simulink model "indmotorwithcc"  (R2021b)
settings: Solver=FixedStepAuto  StartTime=0.0  StopTime=1  FixedStep=1e-5  MinStep=1e-100  RelTol=1e-3
values from neighbouring files (symbols this model uses):
  Vdc = 300    [Induction_motor_parameter.m]
undefined symbols (not defined in the file or in its folder): A, alpha, Iqse_rated, Jm, Kac, Kas, Kic, Kpc, Kps, Kt, Lam_dre_rated, Lm, Lr, Ls, p, pp, Rr, Rs, sigma, Te_rated, Vs_rated, Ws
settings Model: Creator=lhjoon  LastModifiedBy=jun
settings SolverCC: AlgebraicLoopSolver=TrustRegion
settings DataIOCC: SaveFormat=Array  ReturnWorkspaceOutputs=off
settings DebuggingCC: SFMachineParentedDataDiag=warning
settings SFSimCC: CustomCodeUndefinedFunction=UseInterfaceOnly

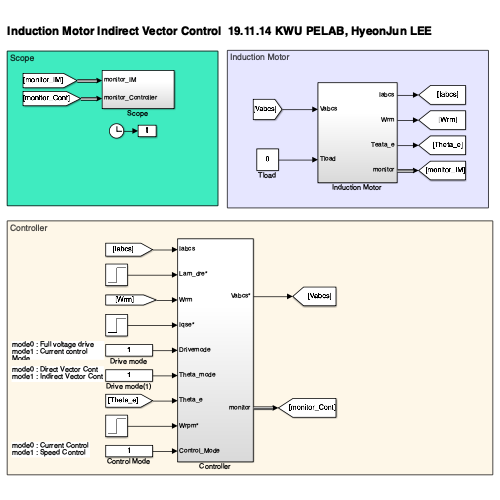
[thumbnail: Simulink's stored preview of the top-level diagram]
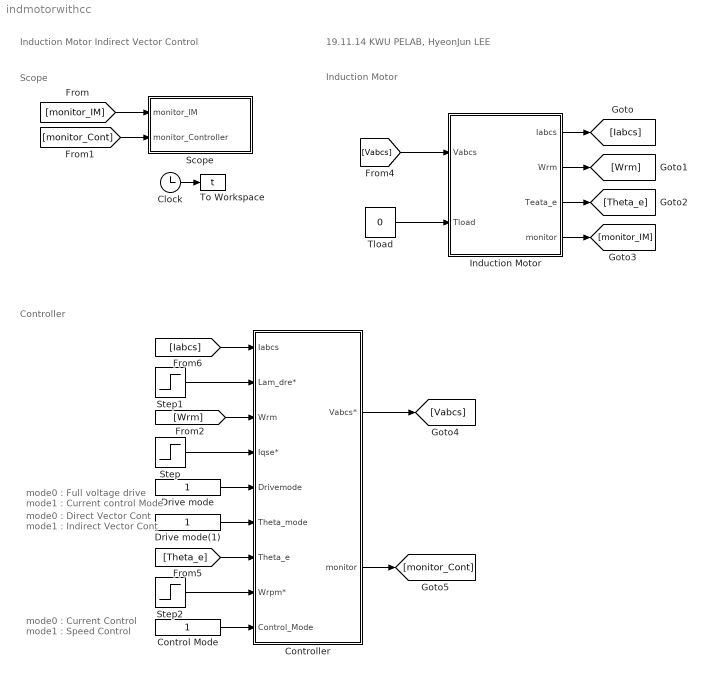
== system indmotorwithcc ==
  note: Controller
  note: mode0 : Full voltage drive
      | mode1 : Current control Mode
  note: Scope
  note: Induction Motor
  note: Induction Motor Indirect Vector Control
  note: mode0 : Direct Vector Cont
      | mode1 : Indirect Vector Cont
  note: 19.11.14 KWU PELAB, HyeonJun LEE
  note: mode0 : Current Control
      | mode1 : Speed Control
  Clock : Clock
  Control Mode : Constant
  Controller : Subsystem
  Drive mode : Constant
  Drive mode(1) : Constant
  Induction Motor : Subsystem
  Scope : Subsystem
  Step : Step  Time=0.2  After=8  SampleTime=0
  Step1 : Step  Time=0.1  After=Lam_dre_rated  SampleTime=0
  Step2 : Step  Time=0.3  After=1500  SampleTime=0
  "Tload " : Constant  Value=0
  To Workspace : ToWorkspace  VariableName=t  SampleTime=-1
  wires:
  Induction Motor/3(Teata_e) -> [Theta_e]
  Induction Motor/1(Iabcs) -> [Iabcs]
  Induction Motor/2(Wrm) -> [Wrm]
  Induction Motor/4(monitor) -> [monitor_IM]
  "Tload "/1 -> Induction Motor/2(Tload)
  Clock/1 -> To Workspace/1
  [monitor_IM] -> Scope/1(monitor_IM)
  [monitor_Cont] -> Scope/2(monitor_Controller)
  Controller/1(Vabcs*) -> [Vabcs]
  [Vabcs] -> Induction Motor/1(Vabcs)
  Drive mode/1 -> Controller/5(Drivemode)
  [Theta_e] -> Controller/7(Theta_e)
  [Iabcs] -> Controller/1(Iabcs)
  [Wrm] -> Controller/3(Wrm)
  Step1/1 -> Controller/2(Lam_dre*)
  Drive mode(1)/1 -> Controller/6(Theta_mode)
  Step/1 -> Controller/4(Iqse*)
  Controller/2(monitor) -> [monitor_Cont]
  Step2/1 -> Controller/8(Wrpm*)
  Control Mode/1 -> Controller/9(Control_Mode)

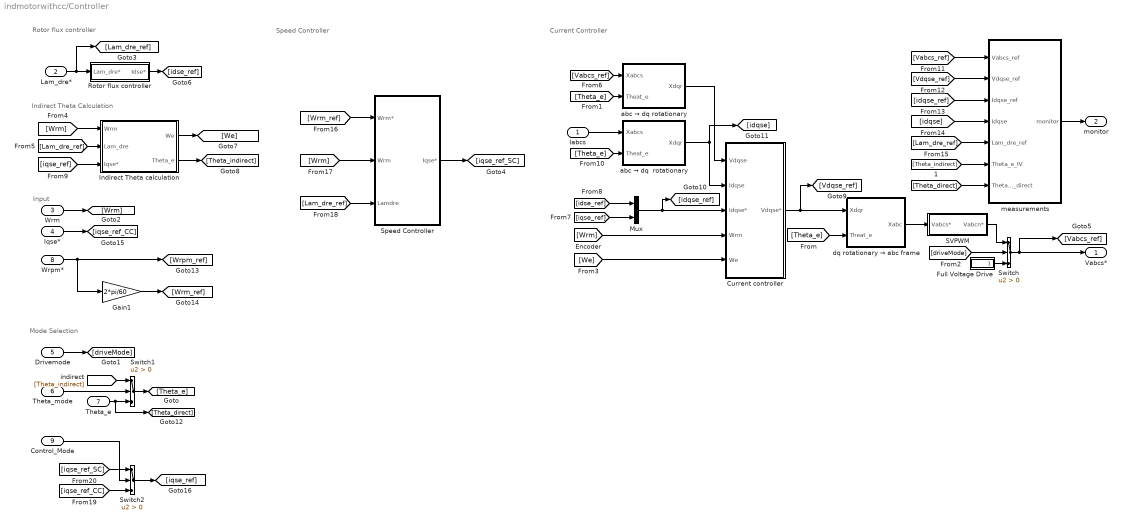
== system indmotorwithcc/Controller ==
  note: Mode Selection
  note: Speed Controller
  note: Current Controller
  note: Input
  note: Indirect Theta Calculation
  note: Rotor flux controller
  Iabcs : Inport
  Lam_dre* : Inport  Port=2
  Wrm : Inport  Port=3
  Iqse* : Inport  Port=4
  Drivemode : Inport  Port=5
  Theta_mode : Inport  Port=6
  Theta_e : Inport  Port=7
  Wrpm* : Inport  Port=8
  Control_Mode : Inport  Port=9
  "Current controller " : Subsystem
  Full Voltage Drive : Subsystem
  Gain1 : Gain  Gain=2*pi/60
  Indirect Theta calculation : Subsystem
  Mux : Mux  Inputs=2
  Rotor flux controller : Subsystem
  SVPWM : Subsystem
  Speed Controller : Subsystem
  Switch : Switch  Criteria=u2 > Threshold
  Switch1 : Switch  Criteria=u2 > Threshold
  Switch2 : Switch  Criteria=u2 > Threshold
  abc → dq  rotationary : Subsystem
  abc → dq rotationary : Subsystem
  dq rotationary → abc frame : Subsystem
  measurements : Subsystem
  Vabcs* : Outport  VectorParamsAs1DForOutWhenUnconnected=off
  monitor : Outport  Port=2  VectorParamsAs1DForOutWhenUnconnected=off
  wires:
  Full Voltage Drive/1(Vabcs) -> Switch/3
  [driveMode] -> Switch/2
  Switch/1 -> Vabcs*/1, [Vabcs_ref]
  dq rotationary → abc frame/1(Xabc) -> SVPWM/1(Vabcs*)
  Iabcs/1 -> abc → dq  rotationary/1(Xabcs)
  abc → dq  rotationary/1(Xdqr) -> [idqse], "Current controller "/2(Idqse)
  [Theta_e] -> dq rotationary → abc frame/2("Theat_e ")
  [Theta_e] -> abc → dq rotationary/2(Theat_e)
  abc → dq rotationary/1(Xdqr) -> "Current controller "/1(Vdqse)
  Drivemode/1 -> [driveMode]
  Wrm/1 -> [Wrm]
  [Wrm] -> "Current controller "/4(Wrm)
  Iqse*/1 -> [iqse_ref_CC]
  [We] -> "Current controller "/5(We)
  Lam_dre*/1 -> [Lam_dre_ref], Rotor flux controller/1(Lam_dre*)
  [Wrm] -> Indirect Theta calculation/1(Wrm)
  [Lam_dre_ref] -> Indirect Theta calculation/2(Lam_dre)
  Mux/1 -> [idqse_ref], "Current controller "/3(Idqse*)
  [Vabcs_ref] -> abc → dq rotationary/1(Xabcs)
  [idse_ref] -> Mux/1
  [iqse_ref] -> Mux/2
  Rotor flux controller/1(Idse*) -> [idse_ref]
  [iqse_ref] -> Indirect Theta calculation/3(Iqse*)
  Indirect Theta calculation/1(We) -> [We]
  Indirect Theta calculation/2(Theta_e) -> [Theta_indirect]
  Theta_mode/1 -> Switch1/2
  Switch1/1 -> [Theta_e]
  [Theta_indirect] -> Switch1/1
  Theta_e/1 -> [Theta_direct], Switch1/3
  [Theta_e] -> abc → dq  rotationary/2(Theat_e)
  measurements/1(monitor) -> monitor/1
  [Vabcs_ref] -> measurements/1(Vabcs_ref)
  "Current controller "/1(Vdqse*) -> [Vdqse_ref], dq rotationary → abc frame/1(Xdqr)
  [Vdqse_ref] -> measurements/2(Vdqse_ref)
  [idqse_ref] -> measurements/3(Idqse_ref)
  SVPWM/1(Vabcn*) -> Switch/1
  [idqse] -> measurements/4(Idqse)
  [Theta_indirect] -> measurements/6(Theta_e_IV)
  [Lam_dre_ref] -> measurements/5(Lam_dre_ref)
  [Theta_direct] -> measurements/7(Theta_e_direct)
  Wrpm*/1 -> Gain1/1, [Wrpm_ref]
  Gain1/1 -> [Wrm_ref]
  [Wrm_ref] -> Speed Controller/1(Wrm*)
  [Wrm] -> Speed Controller/2("Wrm ")
  [Lam_dre_ref] -> Speed Controller/3(Lamdre)
  Speed Controller/1(Iqse*) -> [iqse_ref_SC]
  Control_Mode/1 -> Switch2/2
  [iqse_ref_SC] -> Switch2/1
  [iqse_ref_CC] -> Switch2/3
  Switch2/1 -> [iqse_ref]

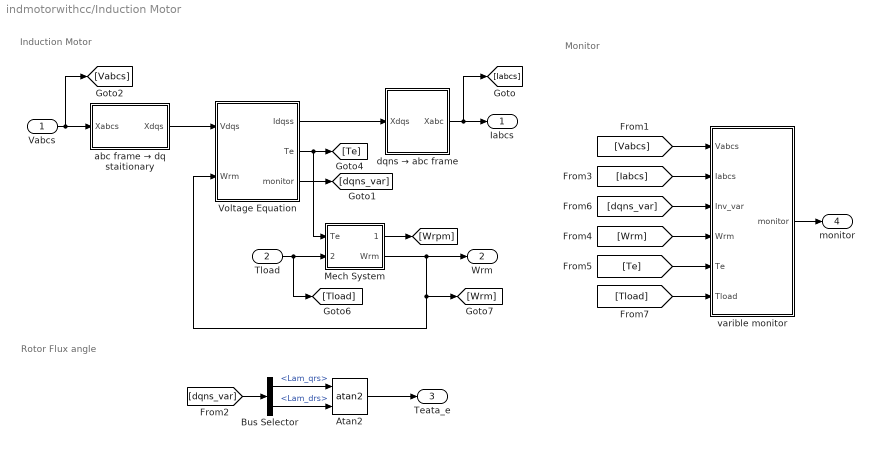
== system indmotorwithcc/Induction Motor ==
  note: Monitor
  note: Rotor Flux angle
  note: Induction Motor
  Vabcs : Inport
  Tload : Inport  Port=2
  Atan2 : Trigonometry  Operator=atan2
  Bus Selector : BusSelector  OutputSignals=Lam_qrs,Lam_drs
  Mech System : Subsystem
  Voltage Equation : Subsystem
  abc frame → dq staitionary : Subsystem
  dqns → abc frame : Subsystem
  varible monitor : Subsystem
  Iabcs : Outport  VectorParamsAs1DForOutWhenUnconnected=off
  Wrm : Outport  Port=2  VectorParamsAs1DForOutWhenUnconnected=off
  Teata_e : Outport  Port=3  VectorParamsAs1DForOutWhenUnconnected=off
  monitor : Outport  Port=4  VectorParamsAs1DForOutWhenUnconnected=off
  wires:
  Voltage Equation/3(monitor) -> [dqns_var]
  Voltage Equation/1(Idqss) -> dqns → abc frame/1(Xdqs)
  Bus Selector/2 -> Atan2/2  "<Lam_drs>"
  Atan2/1 -> Teata_e/1
  Bus Selector/1 -> Atan2/1  "<Lam_qrs>"
  Mech System/1(Wrpm) -> [Wrpm]
  Voltage Equation/2(Te) -> Mech System/1(Te), [Te]
  abc frame → dq staitionary/1(Xdqs) -> Voltage Equation/1(Vdqs)
  [dqns_var] -> Bus Selector/1
  Vabcs/1 -> [Vabcs], abc frame → dq staitionary/1(Xabcs)
  dqns → abc frame/1(Xabc) -> [Iabcs], Iabcs/1
  [Tload] -> varible monitor/6(Tload)
  [Te] -> varible monitor/5(Te)
  [Wrm] -> varible monitor/4(Wrm)
  [dqns_var] -> varible monitor/3(Inv_var)
  [Iabcs] -> varible monitor/2(Iabcs)
  [Vabcs] -> varible monitor/1(Vabcs)
  varible monitor/1(monitor) -> monitor/1
  Tload/1 -> [Tload], Mech System/2(TLoad)
  Mech System/2(Wrm) -> Voltage Equation/2(Wrm), [Wrm], Wrm/1

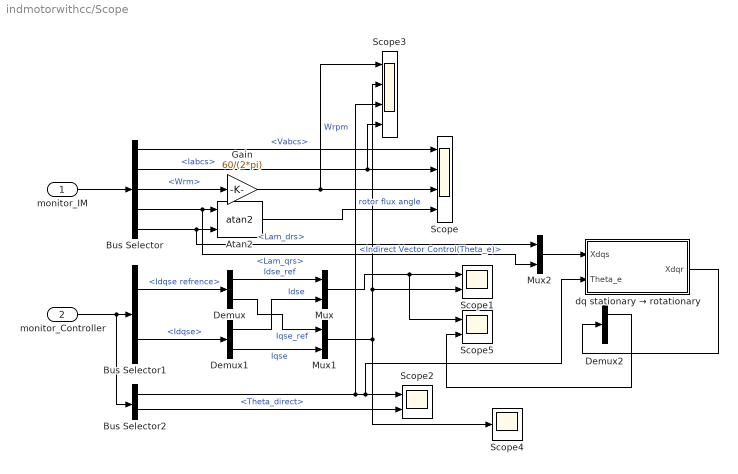
== system indmotorwithcc/Scope ==
  monitor_IM : Inport
  monitor_Controller : Inport  Port=2
  Atan2 : Trigonometry  Operator=atan2
  Bus Selector : BusSelector  OutputSignals=Electrical.3-phase.Vabcs,Electrical.3-phase.Iabcs,Mechanical.Wrm,Electrical.Stationary refrence frame.Lam_qrs,Electrical.Stationary refrence frame.Lam_drs
  Bus Selector1 : BusSelector  OutputSignals=Reference.Idqse refrence,Reference.Idqse
  Bus Selector2 : BusSelector  OutputSignals=Indirect Vector Control(Theta_e),Theta_direct
  Demux : Demux  Outputs=2
  Demux1 : Demux  Outputs=2
  Demux2 : Demux  Outputs=2
  Gain : Gain  Gain=60/(2*pi)
  Mux : Mux  Inputs=2
  Mux1 : Mux  Inputs=2
  Mux2 : Mux  Inputs=2
  Scope : Scope  NumInputPorts=4
  Scope1 : Scope  NumInputPorts=2
  Scope2 : Scope  NumInputPorts=2
  Scope3 : Scope  NumInputPorts=4
  Scope4 : Scope
  Scope5 : Scope  NumInputPorts=2
  dq stationary → rotationary : Subsystem
  wires:
  monitor_IM/1 -> Bus Selector/1
  Bus Selector/1 -> Scope/1  "<Vabcs>"
  Bus Selector/2 -> Scope3/4, Scope/2  "<Iabcs>"
  Bus Selector/3 -> Gain/1  "<Wrm>"
  Bus Selector/4 -> Mux2/2, Atan2/1  "<Lam_qrs>"
  Bus Selector/5 -> Mux2/1, Atan2/2  "<Lam_drs>"
  Atan2/1 -> Scope/4  "rotor flux angle"
  Gain/1 -> Scope3/1, Scope/3  "Wrpm"
  monitor_Controller/1 -> Bus Selector2/1, Bus Selector1/1
  Bus Selector1/1 -> Demux/1  "<Idqse refrence>"
  Bus Selector1/2 -> Demux1/1  "<Idqse>"
  Demux/1 -> Mux/1  "Idse_ref"
  Demux1/1 -> Mux/2  "Idse"
  Demux/2 -> Mux1/1  "Iqse_ref"
  Demux1/2 -> Mux1/2  "Iqse"
  Mux/1 -> Scope5/1, Scope1/1
  Mux1/1 -> Scope3/2, Scope1/2, Scope4/1
  Bus Selector2/1 -> Scope3/3, dq stationary → rotationary/2(Theta_e), Scope2/1  "<Indirect Vector Control(Theta_e)>"
  Bus Selector2/2 -> Scope2/2  "<Theta_direct>"
  Mux2/1 -> dq stationary → rotationary/1(Xdqs)
  dq stationary → rotationary/1(Xdqr) -> Demux2/1
  Demux2/1 -> Scope5/2

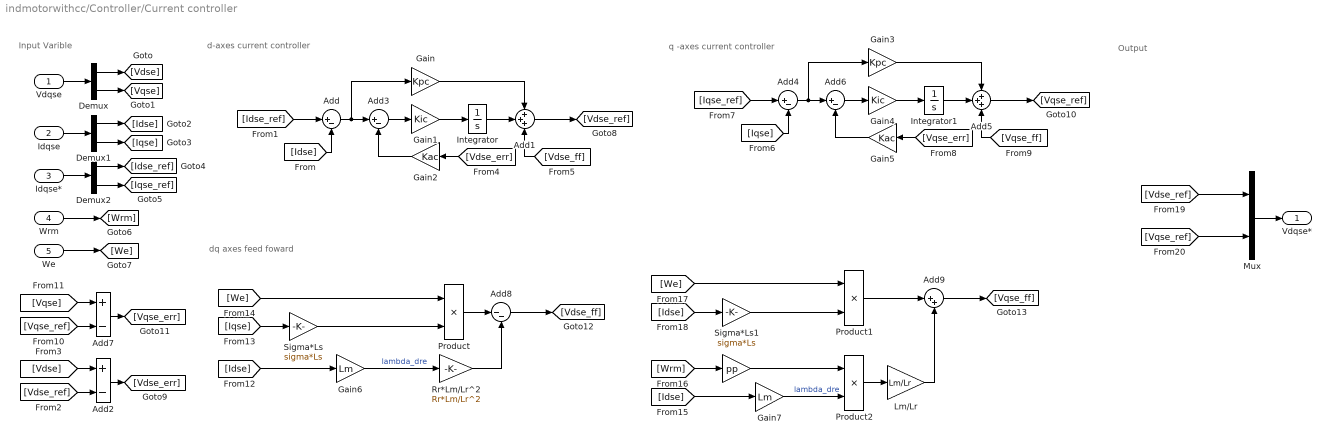
== system indmotorwithcc/Controller/Current controller  ==
  note: Output
  note: q -axes current controller
  note: d-axes current controller
  note: dq axes feed foward
  note: Input Varible
  Vdqse : Inport
  Idqse : Inport  Port=2
  Idqse* : Inport  Port=3
  Wrm : Inport  Port=4
  We : Inport  Port=5
  " " : Gain  Gain=pp
  Add{,3..4,6} (4 alike) : Sum  Inputs=|+-
  Add1 : Sum  Inputs=+++
  Add2 : Sum  Inputs=+-
  Add5 : Sum  Inputs=+++
  Add7 : Sum  Inputs=+-
  Add8 : Sum  Inputs=|--
  Add9 : Sum  Inputs=|++
  Demux : Demux  Outputs=2
  Demux1 : Demux  Outputs=2
  Demux2 : Demux  Outputs=2
  Gain : Gain  Gain=Kpc
  Gain1 : Gain  Gain=Kic
  Gain2 : Gain  Gain=Kac
  Gain3 : Gain  Gain=Kpc
  Gain4 : Gain  Gain=Kic
  Gain5 : Gain  Gain=Kac
  Gain6 : Gain  Gain=Lm
  Gain7 : Gain  Gain=Lm
  Integrator : Integrator
  Integrator1 : Integrator
  Lm/Lr : Gain  Gain=Lm/Lr
  Mux : Mux  Inputs=2
  Product : Product
  Product1 : Product
  Product2 : Product
  "Rr*Lm/Lr^2 " : Gain  Gain=Rr*Lm/Lr^2
  Sigma*Ls : Gain  Gain=sigma*Ls
  Sigma*Ls1 : Gain  Gain=sigma*Ls
  Vdqse* : Outport  VectorParamsAs1DForOutWhenUnconnected=off
  wires:
  Vdqse/1 -> Demux/1
  Demux/1 -> [Vdse]
  Demux/2 -> [Vqse]
  Demux1/1 -> [Idse]
  Idqse/1 -> Demux1/1
  Demux1/2 -> [Iqse]
  Demux2/1 -> [Idse_ref]
  Demux2/2 -> [Iqse_ref]
  Idqse*/1 -> Demux2/1
  Wrm/1 -> [Wrm]
  We/1 -> [We]
  [Idse] -> Add/2
  [Idse_ref] -> Add/1
  Add/1 -> Add3/1, Gain/1
  Gain1/1 -> Integrator/1
  Integrator/1 -> Add1/2
  Gain/1 -> Add1/1
  Add1/1 -> [Vdse_ref]
  [Vdse] -> Add2/1
  [Vdse_ref] -> Add2/2
  Add2/1 -> [Vdse_err]
  Add3/1 -> Gain1/1
  [Vdse_err] -> Gain2/1
  Gain2/1 -> Add3/2
  [Vdse_ff] -> Add1/3
  [Vqse_err] -> Gain5/1
  Gain5/1 -> Add6/2
  [Iqse] -> Add4/2
  Gain4/1 -> Integrator1/1
  Add6/1 -> Gain4/1
  Add4/1 -> Add6/1, Gain3/1
  Add5/1 -> [Vqse_ref]
  Gain3/1 -> Add5/1
  [Iqse_ref] -> Add4/1
  Integrator1/1 -> Add5/2
  [Vqse_ff] -> Add5/3
  [Vqse_ref] -> Add7/2
  Add7/1 -> [Vqse_err]
  [Vqse] -> Add7/1
  Add8/1 -> [Vdse_ff]
  "Rr*Lm/Lr^2 "/1 -> Add8/2
  [Idse] -> Gain6/1
  Gain6/1 -> "Rr*Lm/Lr^2 "/1  "lambda_dre"
  Product/1 -> Add8/1
  [Iqse] -> Sigma*Ls/1
  Sigma*Ls/1 -> Product/2
  [We] -> Product/1
  Product1/1 -> Add9/1
  Add9/1 -> [Vqse_ff]
  Lm/Lr/1 -> Add9/2
  Product2/1 -> Lm/Lr/1
  [Idse] -> Gain7/1
  Gain7/1 -> Product2/2  "lambda_dre"
  [Wrm] -> " "/1
  " "/1 -> Product2/1
  [We] -> Product1/1
  Sigma*Ls1/1 -> Product1/2
  [Idse] -> Sigma*Ls1/1
  Mux/1 -> Vdqse*/1
  [Vdse_ref] -> Mux/1
  [Vqse_ref] -> Mux/2

== system indmotorwithcc/Controller/Full Voltage Drive ==
  note: Full Voltage (RMS 220V)
  Mux : Mux  Inputs=3
  Vas : Sin  Amplitude=Vs_rated  Frequency=Ws  SampleTime=0
  Vbs : Sin  Amplitude=Vs_rated  Frequency=Ws  Phase=-2/3*pi  SampleTime=0
  Vcs : Sin  Amplitude=Vs_rated  Frequency=Ws  Phase=2/3*pi  SampleTime=0
  Vabcs : Outport  VectorParamsAs1DForOutWhenUnconnected=off
  wires:
  Vcs/1 -> Mux/3
  Vas/1 -> Mux/1
  Mux/1 -> Vabcs/1
  Vbs/1 -> Mux/2

== system indmotorwithcc/Controller/Indirect Theta calculation ==
  Wrm : Inport
  Lam_dre : Inport  Port=2
  Iqse* : Inport  Port=3
  Add : Sum  Inputs=|++
  Divide : Product  Inputs=*/
  Gain : Gain  Gain=pp
  Integrator : Subsystem
  Rr*Lm/Lr : Gain  Gain=Lm/Lr*Rr
  Saturation4 : Saturate  UpperLimit=inf  LowerLimit=1e-04
  We : Outport  VectorParamsAs1DForOutWhenUnconnected=off
  Theta_e : Outport  Port=2  VectorParamsAs1DForOutWhenUnconnected=off
  wires:
  Iqse*/1 -> Rr*Lm/Lr/1
  Lam_dre/1 -> Saturation4/1
  Saturation4/1 -> Divide/2
  Rr*Lm/Lr/1 -> Divide/1
  Divide/1 -> Add/1  "Wsl"
  Wrm/1 -> Gain/1
  Gain/1 -> Add/2  "Wr"
  Add/1 -> Integrator/1(We), We/1
  Integrator/1(Theta_e) -> Theta_e/1

== system indmotorwithcc/Controller/Rotor flux controller ==
  Lam_dre* : Inport
  Gain : Gain  Gain=1/Lm
  Idse* : Outport  VectorParamsAs1DForOutWhenUnconnected=off
  wires:
  Gain/1 -> Idse*/1
  Lam_dre*/1 -> Gain/1

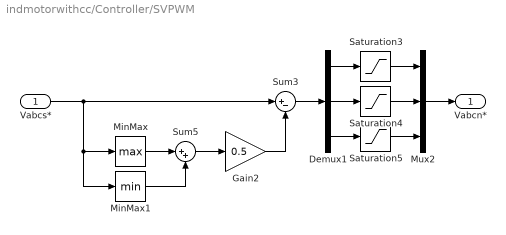
== system indmotorwithcc/Controller/SVPWM ==
  Vabcs* : Inport
  Demux1 : Demux  Outputs=3
  Gain2 : Gain  Gain=0.5
  MinMax : MinMax  Function=max
  MinMax1 : MinMax
  Mux2 : Mux  Inputs=3
  Saturation3 : Saturate  UpperLimit=Vdc/2  LowerLimit=-Vdc/2
  Saturation4 : Saturate  UpperLimit=Vdc/2  LowerLimit=-Vdc/2
  Saturation5 : Saturate  UpperLimit=Vdc/2  LowerLimit=-Vdc/2
  Sum3 : Sum  Inputs=|+-
  Sum5 : Sum  Inputs=|++
  Vabcn* : Outport  VectorParamsAs1DForOutWhenUnconnected=off
  wires:
  Vabcs*/1 -> Sum3/1, MinMax1/1, MinMax/1
  MinMax/1 -> Sum5/1
  Sum5/1 -> Gain2/1
  MinMax1/1 -> Sum5/2
  Gain2/1 -> Sum3/2
  Demux1/1 -> Saturation3/1
  Demux1/2 -> Saturation4/1
  Demux1/3 -> Saturation5/1
  Sum3/1 -> Demux1/1
  Saturation3/1 -> Mux2/1
  Saturation4/1 -> Mux2/2
  Saturation5/1 -> Mux2/3
  Mux2/1 -> Vabcn*/1

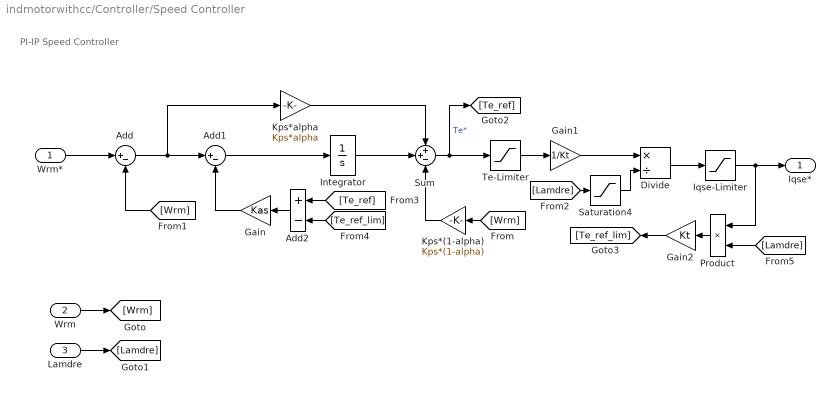
== system indmotorwithcc/Controller/Speed Controller ==
  note: PI-IP Speed Controller
  Wrm* : Inport
  "Wrm " : Inport  Port=2
  Lamdre : Inport  Port=3
  Add : Sum  Inputs=|+-
  Add1 : Sum  Inputs=|+-
  Add2 : Sum  Inputs=+-
  Divide : Product  Inputs=*/
  Gain : Gain  Gain=Kas
  Gain1 : Gain  Gain=1/Kt
  Gain2 : Gain  Gain=Kt
  Integrator : Integrator
  Iqse-Limiter : Saturate  UpperLimit=Iqse_rated  LowerLimit=-Iqse_rated
  Kps*(1-alpha) : Gain  Gain=Kps*(1-alpha)
  Kps*alpha : Gain  Gain=Kps*alpha
  Product : Product
  Saturation4 : Saturate  UpperLimit=inf  LowerLimit=1e-04
  Sum : Sum  Inputs=++-
  Te-Limiter : Saturate  UpperLimit=Te_rated  LowerLimit=-Te_rated
  Iqse* : Outport  VectorParamsAs1DForOutWhenUnconnected=off
  wires:
  Wrm*/1 -> Add/1
  "Wrm "/1 -> [Wrm]
  Lamdre/1 -> [Lamdre]
  Add/1 -> Kps*alpha/1, Add1/1
  Gain/1 -> Add1/2
  Add1/1 -> Integrator/1
  Integrator/1 -> Sum/2
  Kps*(1-alpha)/1 -> Sum/3
  Kps*alpha/1 -> Sum/1
  [Wrm] -> Add/2
  [Wrm] -> Kps*(1-alpha)/1
  Add2/1 -> Gain/1
  Sum/1 -> Te-Limiter/1, [Te_ref]  "Te*"
  Te-Limiter/1 -> Gain1/1
  Gain1/1 -> Divide/1
  Divide/1 -> Iqse-Limiter/1
  Iqse-Limiter/1 -> Iqse*/1, Product/1
  [Te_ref] -> Add2/1
  [Te_ref_lim] -> Add2/2
  [Lamdre] -> Product/2
  Gain2/1 -> [Te_ref_lim]
  Product/1 -> Gain2/1
  Saturation4/1 -> Divide/2
  [Lamdre] -> Saturation4/1

== system indmotorwithcc/Controller/abc → dq  rotationary ==
  Xabcs : Inport
  Theat_e : Inport  Port=2
  abc frame → dq staitionary : Subsystem
  dq stationary → rotationary : Subsystem
  Xdqr : Outport  VectorParamsAs1DForOutWhenUnconnected=off
  wires:
  Xabcs/1 -> abc frame → dq staitionary/1(Xabcs)
  abc frame → dq staitionary/1(Xdqs) -> dq stationary → rotationary/1(Xdqs)
  Theat_e/1 -> dq stationary → rotationary/2(Theta_e)
  dq stationary → rotationary/1(Xdqr) -> Xdqr/1

== system indmotorwithcc/Controller/abc → dq rotationary ==
  Xabcs : Inport
  Theat_e : Inport  Port=2
  abc frame → dq staitionary : Subsystem
  dq stationary → rotationary : Subsystem
  Xdqr : Outport  VectorParamsAs1DForOutWhenUnconnected=off
  wires:
  Xabcs/1 -> abc frame → dq staitionary/1(Xabcs)
  abc frame → dq staitionary/1(Xdqs) -> dq stationary → rotationary/1(Xdqs)
  Theat_e/1 -> dq stationary → rotationary/2(Theta_e)
  dq stationary → rotationary/1(Xdqr) -> Xdqr/1

== system indmotorwithcc/Controller/dq rotationary → abc frame ==
  Xdqr : Inport
  "Theat_e " : Inport  Port=2
  dq rotatinoary → dq stationary : Subsystem
  dq stationary → abc frame : Subsystem
  Xabc : Outport  VectorParamsAs1DForOutWhenUnconnected=off
  wires:
  "Theat_e "/1 -> dq rotatinoary → dq stationary/2(Theta_e)
  Xdqr/1 -> dq rotatinoary → dq stationary/1(Xdqr)
  dq rotatinoary → dq stationary/1(Xdqs) -> dq stationary → abc frame/1(Xdqs)
  dq stationary → abc frame/1(Xabc) -> Xabc/1

== system indmotorwithcc/Controller/measurements ==
  Vabcs_ref : Inport
  Vdqse_ref : Inport  Port=2
  Idqse_ref : Inport  Port=3
  Idqse : Inport  Port=4
  Lam_dre_ref : Inport  Port=5
  Theta_e_IV : Inport  Port=6
  Theta_e_direct : Inport  Port=7
  Bus Creator1 : BusCreator  Inputs=2
  Bus Creator2 : BusCreator  Inputs=4
  Bus Creator4 : BusCreator  Inputs=3
  monitor : Outport  VectorParamsAs1DForOutWhenUnconnected=off
  wires:
  Theta_e_IV/1 -> Bus Creator4/2  "Indirect Vector Control(Theta_e)"
  Idqse_ref/1 -> Bus Creator2/2  "Idqse refrence"
  Bus Creator4/1 -> monitor/1
  Bus Creator2/1 -> Bus Creator4/1  "Reference"
  Bus Creator1/1 -> Bus Creator2/1  "Voltage reference"
  Lam_dre_ref/1 -> Bus Creator2/4  "Lam_dre_ref"
  Vdqse_ref/1 -> Bus Creator1/2  "Vdqse_ref"
  Vabcs_ref/1 -> Bus Creator1/1  "Vabcs_ref"
  Idqse/1 -> Bus Creator2/3  "Idqse"
  Theta_e_direct/1 -> Bus Creator4/3  "Theta_direct"

== system indmotorwithcc/Induction Motor/Mech System ==
  note: Mech System
  Te : Inport
  TLoad : Inport  Port=2
  Add : Sum  Inputs=+-
  Gain : Gain  Gain=1/Jm
  Gain1 : Gain  Gain=60/(2*pi)
  Integrator : Integrator
  Wrpm : Outport  VectorParamsAs1DForOutWhenUnconnected=off
  Wrm : Outport  Port=2  VectorParamsAs1DForOutWhenUnconnected=off
  wires:
  Integrator/1 -> Gain1/1, Wrm/1
  Gain/1 -> Integrator/1
  Te/1 -> Add/1
  Add/1 -> Gain/1
  TLoad/1 -> Add/2
  Gain1/1 -> Wrpm/1

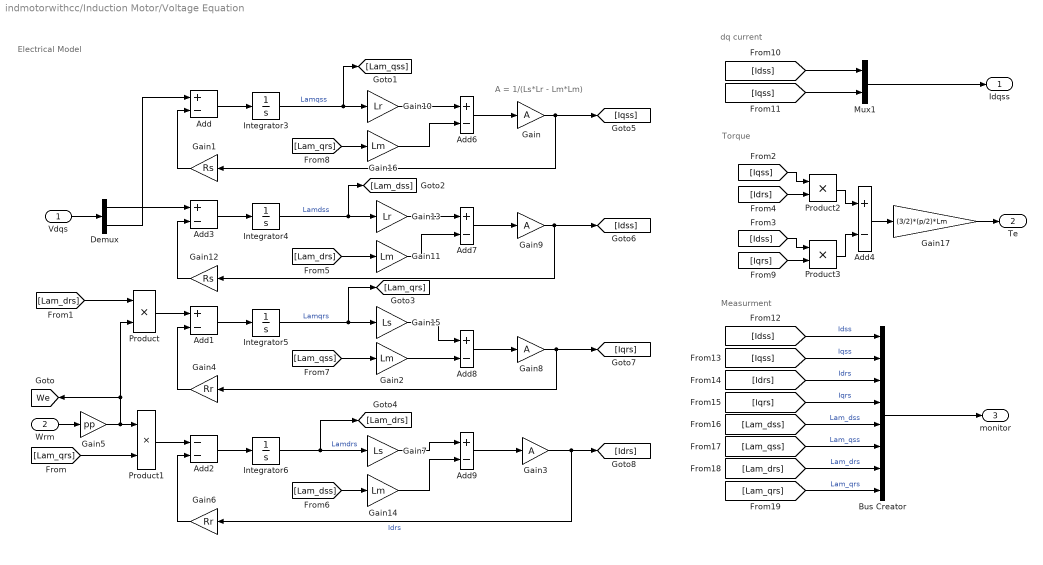
== system indmotorwithcc/Induction Motor/Voltage Equation ==
  note: Measurment
  note: dq current
  note: Torque
  note: Electrical Model
  note: A = 1/(Ls*Lr - Lm*Lm)
  Vdqs : Inport
  Wrm : Inport  Port=2
  Add{,1,3..4,6..9} (8 alike) : Sum  Inputs=+-
  Add2 : Sum  Inputs=--
  Bus Creator : BusCreator  Inputs=8
  Demux : Demux  Outputs=2
  Gain{,3,8..9} (4 alike) : Gain  Gain=A
  Gain1 : Gain  Gain=Rs
  Gain10 : Gain  Gain=Lr
  Gain{2,11,14,16} (4 alike) : Gain  Gain=Lm
  Gain12 : Gain  Gain=Rs
  Gain13 : Gain  Gain=Lr
  Gain15 : Gain  Gain=Ls
  Gain17 : Gain  Gain=(3/2)*(p/2)*Lm
  Gain4 : Gain  Gain=Rr
  Gain5 : Gain  Gain=pp
  Gain6 : Gain  Gain=Rr
  Gain7 : Gain  Gain=Ls
  Integrator{3..6} (4 alike) : Integrator
  Mux1 : Mux  Inputs=2
  Product{,1..3} (4 alike) : Product
  Idqss : Outport  VectorParamsAs1DForOutWhenUnconnected=off
  Te : Outport  Port=2  VectorParamsAs1DForOutWhenUnconnected=off
  monitor : Outport  Port=3  VectorParamsAs1DForOutWhenUnconnected=off
  tag scope: We=global
  wires:
  Gain/1 -> Gain1/1, [Iqss]
  Wrm/1 -> Gain5/1
  Integrator3/1 -> [Lam_qss], Gain10/1  "Lamqss"
  Integrator4/1 -> [Lam_dss], Gain13/1  "Lamdss"
  Integrator5/1 -> [Lam_qrs], Gain15/1  "Lamqrs"
  Integrator6/1 -> [Lam_drs], Gain7/1  "Lamdrs"
  Gain9/1 -> Gain12/1, [Idss]
  Gain8/1 -> [Iqrs], Gain4/1
  Gain3/1 -> [Idrs], Gain6/1  "Idrs"
  Add6/1 -> Gain/1
  Add7/1 -> Gain9/1
  Add8/1 -> Gain8/1
  Add9/1 -> Gain3/1
  Gain10/1 -> Add6/1
  Add/1 -> Integrator3/1
  Gain1/1 -> Add/2
  Add1/1 -> Integrator5/1
  Gain4/1 -> Add1/2
  Product/1 -> Add1/1
  Gain5/1 -> Product/2, [We], Product1/1
  Add2/1 -> Integrator6/1
  Gain6/1 -> Add2/2
  Gain7/1 -> Add9/1
  Add3/1 -> Integrator4/1
  Gain12/1 -> Add3/2
  Gain13/1 -> Add7/1
  Product1/1 -> Add2/1
  Demux/2 -> Add/1
  Gain17/1 -> Te/1
  Add4/1 -> Gain17/1
  Product2/1 -> Add4/1
  Product3/1 -> Add4/2
  [Lam_qrs] -> Product1/2
  [Lam_drs] -> Product/1
  [Iqss] -> Product2/1
  [Idss] -> Product3/1
  [Iqrs] -> Product3/2
  Gain11/1 -> Add7/2
  [Lam_drs] -> Gain11/1
  [Lam_dss] -> Gain14/1
  Gain16/1 -> Add6/2
  [Lam_qss] -> Gain2/1
  Gain15/1 -> Add8/1
  Gain2/1 -> Add8/2
  [Lam_qrs] -> Gain16/1
  [Idrs] -> Product2/2
  Gain14/1 -> Add9/2
  [Idss] -> Mux1/1
  [Iqss] -> Mux1/2
  Mux1/1 -> Idqss/1
  [Idss] -> Bus Creator/1  "Idss"
  [Iqss] -> Bus Creator/2  "Iqss"
  [Idrs] -> Bus Creator/3  "Idrs"
  [Iqrs] -> Bus Creator/4  "Iqrs"
  [Lam_dss] -> Bus Creator/5  "Lam_dss"
  [Lam_qss] -> Bus Creator/6  "Lam_qss"
  [Lam_drs] -> Bus Creator/7  "Lam_drs"
  [Lam_qrs] -> Bus Creator/8  "Lam_qrs"
  Bus Creator/1 -> monitor/1
  Vdqs/1 -> Demux/1
  Demux/1 -> Add3/1

== system indmotorwithcc/Induction Motor/abc frame → dq staitionary ==
  Xabcs : Inport
  Add : Sum  Inputs=+--
  Add1 : Sum  Inputs=+-
  Demux : Demux  Outputs=3
  Gain : Gain  Gain=2
  Gain1 : Gain  Gain=1/3
  Gain2 : Gain  Gain=1/sqrt(3)
  Mux : Mux  Inputs=2
  Xdqs : Outport  VectorParamsAs1DForOutWhenUnconnected=off
  wires:
  Demux/1 -> Gain/1
  Gain/1 -> Add/1
  Demux/2 -> Add1/1, Add/2
  Demux/3 -> Add1/2, Add/3
  Add/1 -> Gain1/1
  Gain1/1 -> Mux/1
  Gain2/1 -> Mux/2
  Add1/1 -> Gain2/1
  Mux/1 -> Xdqs/1
  Xabcs/1 -> Demux/1

== system indmotorwithcc/Induction Motor/dqns → abc frame ==
  Xdqs : Inport
  Add : Sum  Inputs=-+
  Add1 : Sum  Inputs=--
  Demux : Demux  Outputs=2
  Gain : Gain  Gain=1/2
  Gain1 : Gain  Gain=sqrt(3)/2
  Mux : Mux  Inputs=3
  Xabc : Outport  VectorParamsAs1DForOutWhenUnconnected=off
  wires:
  Demux/1 -> Mux/1, Gain/1
  Add/1 -> Mux/2
  Add1/1 -> Mux/3
  Demux/2 -> Gain1/1
  Gain1/1 -> Add1/2, Add/2
  Gain/1 -> Add1/1, Add/1
  Mux/1 -> Xabc/1
  Xdqs/1 -> Demux/1

== system indmotorwithcc/Induction Motor/varible monitor ==
  Vabcs : Inport
  Iabcs : Inport  Port=2
  Inv_var : Inport  Port=3
  Wrm : Inport  Port=4
  Te : Inport  Port=5
  Tload : Inport  Port=6
  Bus Creator1 : BusCreator  Inputs=2
  Bus Creator2 : BusCreator  Inputs=2
  Bus Creator3 : BusCreator  Inputs=4
  Bus Creator4 : BusCreator  Inputs=2
  Gain5 : Gain  Gain=pp
  monitor : Outport  VectorParamsAs1DForOutWhenUnconnected=off
  wires:
  Vabcs/1 -> Bus Creator1/1  "Vabcs"
  Iabcs/1 -> Bus Creator1/2  "Iabcs"
  Bus Creator4/1 -> monitor/1
  Bus Creator1/1 -> Bus Creator2/1  "3-phase"
  Inv_var/1 -> Bus Creator2/2  "Stationary refrence frame"
  Wrm/1 -> Gain5/1, Bus Creator3/1  "Wrm"
  Te/1 -> Bus Creator3/3
  Bus Creator3/1 -> Bus Creator4/2  "Mechanical"
  Bus Creator2/1 -> Bus Creator4/1  "Electrical"
  Gain5/1 -> Bus Creator3/2  "Wr"
  Tload/1 -> Bus Creator3/4

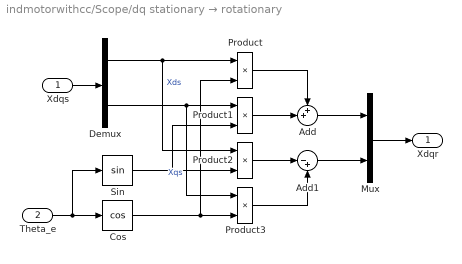
== system indmotorwithcc/Scope/dq stationary → rotationary ==
  Xdqs : Inport
  Theta_e : Inport  Port=2
  Add : Sum  Inputs=++|
  Add1 : Sum  Inputs=|-+
  Cos : Trigonometry  Operator=cos
  Demux : Demux  Outputs=2
  Mux : Mux  Inputs=2
  Product{,1..3} (4 alike) : Product
  Sin : Trigonometry
  Xdqr : Outport  VectorParamsAs1DForOutWhenUnconnected=off
  wires:
  Xdqs/1 -> Demux/1
  Demux/1 -> Product2/1, Product/1  "Xds"
  Demux/2 -> Product3/1, Product1/1  "Xqs"
  Theta_e/1 -> Sin/1, Cos/1
  Cos/1 -> Product3/2, Product/2
  Product/1 -> Add/1
  Product1/1 -> Add/2
  Product2/1 -> Add1/1
  Product3/1 -> Add1/2
  Add1/1 -> Mux/2
  Add/1 -> Mux/1
  Sin/1 -> Product2/2, Product1/2
  Mux/1 -> Xdqr/1

== system indmotorwithcc/Controller/Indirect Theta calculation/Integrator ==
  We : Inport
  Integrator : Integrator
  bound pi : Subsystem
  Theta_e : Outport  VectorParamsAs1DForOutWhenUnconnected=off
  wires:
  We/1 -> Integrator/1
  Integrator/1 -> bound pi/1(theta)
  bound pi/1(bounded_theta) -> Theta_e/1

== system indmotorwithcc/Controller/abc → dq  rotationary/abc frame → dq staitionary ==
  Xabcs : Inport
  Add : Sum  Inputs=+--
  Add1 : Sum  Inputs=+-
  Demux : Demux  Outputs=3
  Gain : Gain  Gain=2
  Gain1 : Gain  Gain=1/3
  Gain2 : Gain  Gain=1/sqrt(3)
  Mux : Mux  Inputs=2
  Xdqs : Outport  VectorParamsAs1DForOutWhenUnconnected=off
  wires:
  Demux/1 -> Gain/1
  Gain/1 -> Add/1
  Demux/2 -> Add1/1, Add/2
  Demux/3 -> Add1/2, Add/3
  Add/1 -> Gain1/1
  Gain1/1 -> Mux/1
  Gain2/1 -> Mux/2
  Add1/1 -> Gain2/1
  Mux/1 -> Xdqs/1
  Xabcs/1 -> Demux/1

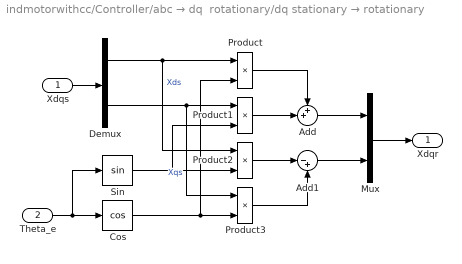
== system indmotorwithcc/Controller/abc → dq  rotationary/dq stationary → rotationary ==
  Xdqs : Inport
  Theta_e : Inport  Port=2
  Add : Sum  Inputs=++|
  Add1 : Sum  Inputs=|-+
  Cos : Trigonometry  Operator=cos
  Demux : Demux  Outputs=2
  Mux : Mux  Inputs=2
  Product{,1..3} (4 alike) : Product
  Sin : Trigonometry
  Xdqr : Outport  VectorParamsAs1DForOutWhenUnconnected=off
  wires:
  Xdqs/1 -> Demux/1
  Demux/1 -> Product2/1, Product/1  "Xds"
  Demux/2 -> Product3/1, Product1/1  "Xqs"
  Theta_e/1 -> Sin/1, Cos/1
  Cos/1 -> Product3/2, Product/2
  Product/1 -> Add/1
  Product1/1 -> Add/2
  Product2/1 -> Add1/1
  Product3/1 -> Add1/2
  Add1/1 -> Mux/2
  Add/1 -> Mux/1
  Sin/1 -> Product2/2, Product1/2
  Mux/1 -> Xdqr/1

== system indmotorwithcc/Controller/abc → dq rotationary/abc frame → dq staitionary ==
  Xabcs : Inport
  Add : Sum  Inputs=+--
  Add1 : Sum  Inputs=+-
  Demux : Demux  Outputs=3
  Gain : Gain  Gain=2
  Gain1 : Gain  Gain=1/3
  Gain2 : Gain  Gain=1/sqrt(3)
  Mux : Mux  Inputs=2
  Xdqs : Outport  VectorParamsAs1DForOutWhenUnconnected=off
  wires:
  Demux/1 -> Gain/1
  Gain/1 -> Add/1
  Demux/2 -> Add1/1, Add/2
  Demux/3 -> Add1/2, Add/3
  Add/1 -> Gain1/1
  Gain1/1 -> Mux/1
  Gain2/1 -> Mux/2
  Add1/1 -> Gain2/1
  Mux/1 -> Xdqs/1
  Xabcs/1 -> Demux/1

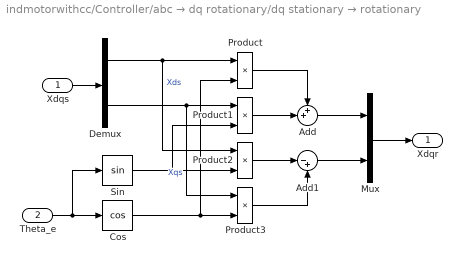
== system indmotorwithcc/Controller/abc → dq rotationary/dq stationary → rotationary ==
  Xdqs : Inport
  Theta_e : Inport  Port=2
  Add : Sum  Inputs=++|
  Add1 : Sum  Inputs=|-+
  Cos : Trigonometry  Operator=cos
  Demux : Demux  Outputs=2
  Mux : Mux  Inputs=2
  Product{,1..3} (4 alike) : Product
  Sin : Trigonometry
  Xdqr : Outport  VectorParamsAs1DForOutWhenUnconnected=off
  wires:
  Xdqs/1 -> Demux/1
  Demux/1 -> Product2/1, Product/1  "Xds"
  Demux/2 -> Product3/1, Product1/1  "Xqs"
  Theta_e/1 -> Sin/1, Cos/1
  Cos/1 -> Product3/2, Product/2
  Product/1 -> Add/1
  Product1/1 -> Add/2
  Product2/1 -> Add1/1
  Product3/1 -> Add1/2
  Add1/1 -> Mux/2
  Add/1 -> Mux/1
  Sin/1 -> Product2/2, Product1/2
  Mux/1 -> Xdqr/1

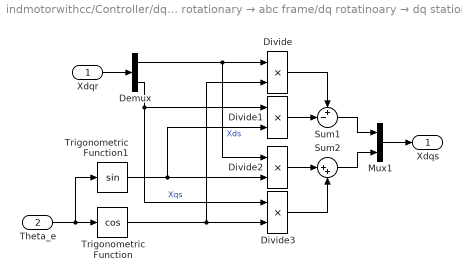
== system indmotorwithcc/Controller/dq rotationary → abc frame/dq rotatinoary → dq stationary ==
  Xdqr : Inport
  Theta_e : Inport  Port=2
  Demux : Demux  Outputs=2
  Divide{,1..3} (4 alike) : Product  Inputs=**
  Mux1 : Mux  Inputs=2
  Sum1 : Sum  Inputs=+-|
  Sum2 : Sum  Inputs=|++
  Trigonometric Function : Trigonometry  Operator=cos
  Trigonometric Function1 : Trigonometry
  Xdqs : Outport  VectorParamsAs1DForOutWhenUnconnected=off
  wires:
  Xdqr/1 -> Demux/1
  Mux1/1 -> Xdqs/1
  Divide3/1 -> Sum2/2
  Sum2/1 -> Mux1/2
  Divide2/1 -> Sum2/1
  Divide/1 -> Sum1/1
  Sum1/1 -> Mux1/1
  Divide1/1 -> Sum1/2
  Theta_e/1 -> Trigonometric Function/1, Trigonometric Function1/1
  Trigonometric Function/1 -> Divide3/2, Divide/2
  Demux/1 -> Divide2/1, Divide/1  "Xds"
  Demux/2 -> Divide3/1, Divide1/1  "Xqs"
  Trigonometric Function1/1 -> Divide2/2, Divide1/2

== system indmotorwithcc/Controller/dq rotationary → abc frame/dq stationary → abc frame ==
  Xdqs : Inport
  Add : Sum  Inputs=-+
  Add1 : Sum  Inputs=--
  Demux : Demux  Outputs=2
  Gain : Gain  Gain=1/2
  Gain1 : Gain  Gain=sqrt(3)/2
  Mux : Mux  Inputs=3
  Xabc : Outport  VectorParamsAs1DForOutWhenUnconnected=off
  wires:
  Demux/1 -> Mux/1, Gain/1
  Add/1 -> Mux/2
  Add1/1 -> Mux/3
  Demux/2 -> Gain1/1
  Gain1/1 -> Add1/2, Add/2
  Gain/1 -> Add1/1, Add/1
  Mux/1 -> Xabc/1
  Xdqs/1 -> Demux/1

== system indmotorwithcc/Controller/Indirect Theta calculation/Integrator/bound pi ==
  theta : Inport
  Gain1 : Gain  Gain=2*pi
  Gain2 : Gain  Gain=1/(2*pi)
  Rounding Function : Rounding  Operator=round
  Subtract : Sum  Inputs=+-
  bounded_theta : Outport  VectorParamsAs1DForOutWhenUnconnected=off
  wires:
  Gain1/1 -> Subtract/2
  theta/1 -> Gain2/1, Subtract/1
  Rounding Function/1 -> Gain1/1
  Gain2/1 -> Rounding Function/1
  Subtract/1 -> bounded_theta/1
